simulink model "Copy_of_Controller"  (R2018b)
settings: configuration reference "control_config" (kept outside this file)
values from neighbouring files (symbols this model uses):
  CONTROL_EXPORT = Simulink.Parameter(CONTROL_EXPORT_VALUE)    [controller_model_init.m]
  CONTROL_PARAM = Simulink.Parameter(CONTROL_PARAM_VALUE)    [controller_model_init.m]
undefined symbols (not defined in the file or in its folder): actuator_cmd, CONTROL_CONST, ControlMode, DiscIntNeverNeededParam, phi_cmd, theta_cmd, timestamp, w_cmd
libraries: simulink x34, FMT_Model_Lib x19
(part 4 of 4)

== system Copy_of_Controller/Controller/MC_Controller/Horizontal_Control/Attitude_Controller/Inner_Loop/Rate_Controller/PID_Controller/I_Control ==
  err : Inport
  reset : Inport  Port=2
  Constant : Constant  Value=[0;0;0]  OutDataTypeStr=single
  Discrete-Time Integrator : DiscreteIntegrator  ExternalReset=level  InitialConditionSource=external  SampleTime=-1  LimitOutput=on  UpperSaturationLimit=max_i  LowerSaturationLimit=min_i  ICPrevOutput=DiscIntNeverNeededParam  ICPrevScaledInput=DiscIntNeverNeededParam
  Multiply : Product  OutDataTypeStr=Inherit: Same as first input
  Mux : Mux  Inputs=3
  gain1 : Constant  Value=p_ki  OutDataTypeStr=single
  gain2 : Constant  Value=q_ki  OutDataTypeStr=single
  gain3 : Constant  Value=r_ki  OutDataTypeStr=single
  i_out : Outport
  wires:
  err/1 -> Multiply/2
  gain2/1 -> Mux/2
  gain1/1 -> Mux/1
  gain3/1 -> Mux/3
  reset/1 -> Discrete-Time Integrator/2
  Constant/1 -> Discrete-Time Integrator/3
  Discrete-Time Integrator/1 -> i_out/1
  Mux/1 -> Multiply/1
  Multiply/1 -> Discrete-Time Integrator/1

== system Copy_of_Controller/Controller/MC_Controller/Horizontal_Control/Attitude_Controller/Inner_Loop/Rate_Controller/PID_Controller/P_Control ==
  err : Inport
  Multiply : Product  OutDataTypeStr=Inherit: Same as first input
  Mux : Mux  Inputs=3
  gain1 : Constant  Value=p_kp  OutDataTypeStr=single
  gain2 : Constant  Value=q_kp  OutDataTypeStr=single
  gain3 : Constant  Value=r_kp  OutDataTypeStr=single
  p_out : Outport
  wires:
  err/1 -> Multiply/2
  gain2/1 -> Mux/2
  Mux/1 -> Multiply/1
  gain1/1 -> Mux/1
  Multiply/1 -> p_out/1
  gain3/1 -> Mux/3

== system Copy_of_Controller/Controller/MC_Controller/Horizontal_Control/Attitude_Controller/Outter_Loop/Attitude_Controller/Error/Bus_Select ==
  INS_Out : Inport
  Bus Selector1 : BusSelector  OutputSignals=phi,theta
  Mux1 : Mux  Inputs=2
  att_est_B_rad : Outport
  wires:
  Bus Selector1/2 -> Mux1/2  "<theta>"
  Bus Selector1/1 -> Mux1/1  "<phi>"
  Mux1/1 -> att_est_B_rad/1
  INS_Out/1 -> Bus Selector1/1

== system Copy_of_Controller/Controller/MC_Controller/Horizontal_Control/Attitude_Controller/Outter_Loop/Attitude_Controller/Sqrt_Root_Controller/Sqrt_Root_Control ==
  error : Inport
  p : Inport  Port=2
  Abs : Abs
  Divide : Product  Inputs=*/
  Divide1 : Product  Inputs=*/
  Gain : Gain  Gain=2  OutDataTypeStr=Inherit: Same as input
  Gain1 : Gain  Gain=-1  OutDataTypeStr=Inherit: Same as input
  Gain2 : Gain  Gain=0.5  OutDataTypeStr=Inherit: Same as input
  Gain3 : Gain  Gain=-1  OutDataTypeStr=Inherit: Same as input
  Logical Operator : Logic  AllPortsSameDT=off  OutDataTypeStr=boolean
  Multiply{,1..3} (4 alike) : Product
  Relational Operator : RelationalOperator  Operator=<=  OutDataTypeStr=boolean  RndMeth=Simplest
  Relational Operator2 : RelationalOperator  OutDataTypeStr=boolean  RndMeth=Simplest
  Saturation Dynamic1 : simulink/Discontinuities/Saturation Dynamic  OutMin=[]  OutMax=[]  OutDataTypeStr=Inherit: Same as second input  OutDataType=fixdt(1, 16)  OutScaling=2^-10  DoSatur=off
  Sign : Signum
  Sqrt : Sqrt  SaturateOnIntegerOverflow=on
  Square : Math  Operator=square  SaturateOnIntegerOverflow=on
  Subtract : Sum  Inputs=+-
  Switch : Switch  Criteria=u2 > Threshold
  const1 : Constant  Value=second_ord_lim  OutDataTypeStr=single
  const2 : Constant  Value=dt  OutDataTypeStr=single
  out : Outport
  wires:
  p/1 -> Multiply/2, Square/1
  const1/1 -> Gain/1, Divide/1
  Square/1 -> Divide/2
  Divide/1 -> Gain2/1, Gain1/1, Relational Operator/2  "linear_dist"
  error/1 -> Abs/1, Multiply/1, Multiply2/2, Sign/1, Relational Operator2/1, Relational Operator/1
  Relational Operator/1 -> Logical Operator/1
  Multiply/1 -> Switch/1
  Switch/1 -> Saturation Dynamic1/2
  Multiply3/1 -> Switch/3
  Gain/1 -> Multiply1/2
  Gain1/1 -> Relational Operator2/2
  Relational Operator2/1 -> Logical Operator/2
  Logical Operator/1 -> Switch/2
  Gain2/1 -> Subtract/2
  Sign/1 -> Multiply3/1, Multiply2/1
  Multiply2/1 -> Subtract/1
  Subtract/1 -> Multiply1/1
  Multiply1/1 -> Sqrt/1
  Sqrt/1 -> Multiply3/2
  Saturation Dynamic1/1 -> out/1
  Abs/1 -> Divide1/1
  const2/1 -> Divide1/2
  Divide1/1 -> Gain3/1, Saturation Dynamic1/1
  Gain3/1 -> Saturation Dynamic1/3

== matlab function Copy_of_Controller/Controller/VTOL_Control_Allocation/VTOL_Control_Allocation/VTOL2/MC_Control_Allocation/R_Remix ==
  data: floating_yaw output; motor_out input; up_lim input; lo_lim input
function floating_yaw = fcn(motor_out, up_lim, lo_lim)

min = single(100);
max = single(-100);
min_index = 0;
max_index = 0;

for i = 1 : 4
    if motor_out(i) < min
       min = motor_out(i);
       min_index = i;
    end
    
    if motor_out(i) > max
       max = motor_out(i);
       max_index = i;
    end
end

if max > up_lim || min < lo_lim
    if (max - up_lim) > (lo_lim - min)
        overrun = up_lim - max;
        if max_index == 3 || max_index == 4
            overrun = -overrun;
        end
    else
        overrun =  lo_lim - min;
        if min_index == 3 || min_index == 4
            overrun = -overrun;
        end
    end
    % we assume effective matrix for yaw is [1 1 -1 -1]
    floating_yaw = single([overrun; overrun; -overrun; -overrun]);
else
    floating_yaw = single(zeros(4,1));
end

== matlab function Copy_of_Controller/Controller/VTOL_Control_Allocation/VTOL_Control_Allocation/VTOL1/MC_Control_Allocation2/MATLAB Function ==
  data: scale output; max input; floating_throttle output; min input; up_lim input; lo_lim input
function [scale, floating_throttle] = fcn(max, min, up_lim, lo_lim)

floating_throttle = single(0);
scale = single(1);

if max > up_lim || min < lo_lim
    if (max - min) > (up_lim - lo_lim)
        floating_throttle = ((up_lim - max) + (lo_lim - min)) / 2;
        scale = (up_lim - lo_lim) / (max - min);
    else
        if max > up_lim
            floating_throttle = up_lim - max;
        else
            floating_throttle = lo_lim - min;
        end
    end
end

== matlab function Copy_of_Controller/Controller/VTOL_Control_Allocation/VTOL_Control_Allocation/VTOL1/MC_Control_Allocation2/MATLAB Function1 ==
  data: floating_yaw output; motor_out input; up_lim input; lo_lim input
function floating_yaw = fcn(motor_out, up_lim, lo_lim)

min = single(100);
max = single(-100);
min_index = 0;
max_index = 0;

for i = 1 : 4
    if motor_out(i) < min
       min = motor_out(i);
       min_index = i;
    end
    
    if motor_out(i) > max
       max = motor_out(i);
       max_index = i;
    end
end

if max > up_lim || min < lo_lim
    if (max - up_lim) > (lo_lim - min)
        diff = up_lim - max;
        if max_index == 3 || max_index == 4
            diff = -diff;
        end
    else
        diff =  lo_lim - min;
        if min_index == 3 || min_index == 4
            diff = -diff;
        end
    end
    floating_yaw = single([diff; diff; -diff; -diff]);
else
    floating_yaw = single(zeros(4,1));
end

== matlab function Copy_of_Controller/Controller/VTOL_Control_Allocation/VTOL_Control_Allocation/VTOL1/MC_Control_Allocation/R_Remix ==
  data: floating_yaw output; motor_out input; up_lim input; lo_lim input
function floating_yaw = fcn(motor_out, up_lim, lo_lim)

min = single(100);
max = single(-100);
min_index = 0;
max_index = 0;

for i = 1 : 4
    if motor_out(i) < min
       min = motor_out(i);
       min_index = i;
    end
    
    if motor_out(i) > max
       max = motor_out(i);
       max_index = i;
    end
end

if max > up_lim || min < lo_lim
    if (max - up_lim) > (lo_lim - min)
        overrun = up_lim - max;
        if max_index == 3 || max_index == 4
            overrun = -overrun;
        end
    else
        overrun =  lo_lim - min;
        if min_index == 3 || min_index == 4
            overrun = -overrun;
        end
    end
    % we assume effective matrix for yaw is [1 1 -1 -1]
    floating_yaw = single([overrun; overrun; -overrun; -overrun]);
else
    floating_yaw = single(zeros(4,1));
end
